simulink model "ColdPT2"  (R2017b)
settings: Solver=FixedStepDiscrete  StartTime=0.0  StopTime=12000  FixedStep=0.5  RelTol=1e-3
values from neighbouring files (symbols this model uses):
  Tt_Reaktor = P2D.Td    [Temperaturverlauf_01-5.m]
libraries: cstblocks x1
settings Model: Creator=arbno  LastModifiedBy=arbno

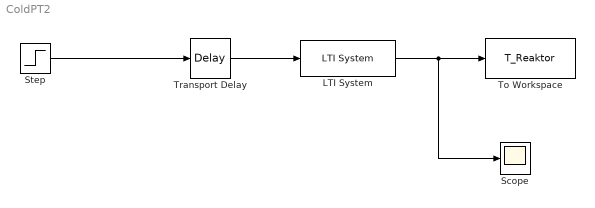
== system ColdPT2 ==
  LTI System : cstblocks/LTI System  sys=G_Z_Reaktor  IC=[]
  Scope : Scope
  Step : Step  After=0.5  SampleTime=0
  To Workspace : ToWorkspace  VariableName=T_Reaktor  SaveFormat=Structure With Time  SampleTime=-1
  Transport Delay : TransportDelay  DelayTime=Tt_Reaktor
  wires:
  LTI System/1 -> Scope/1, To Workspace/1
  Step/1 -> Transport Delay/1
  Transport Delay/1 -> LTI System/1
